simulink model "MRAClecture"  (R2022a)
settings: Solver=VariableStepAuto  StartTime=0.0  StopTime=100  RelTol=1e-3
undefined symbols (not defined in the file): a, a_m, b, b_m, c
settings Model: Creator=edgar  LastModifiedBy=edgar

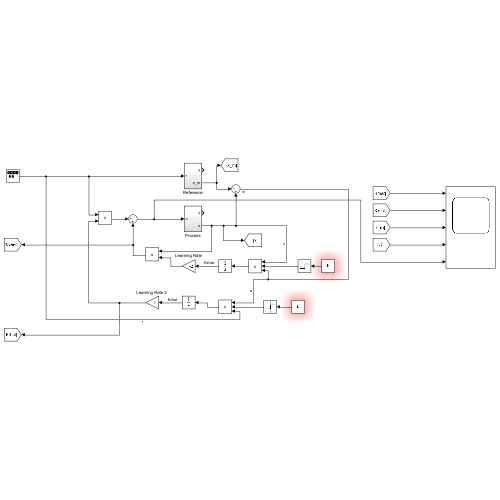
[thumbnail: Simulink's stored preview of the top-level diagram]
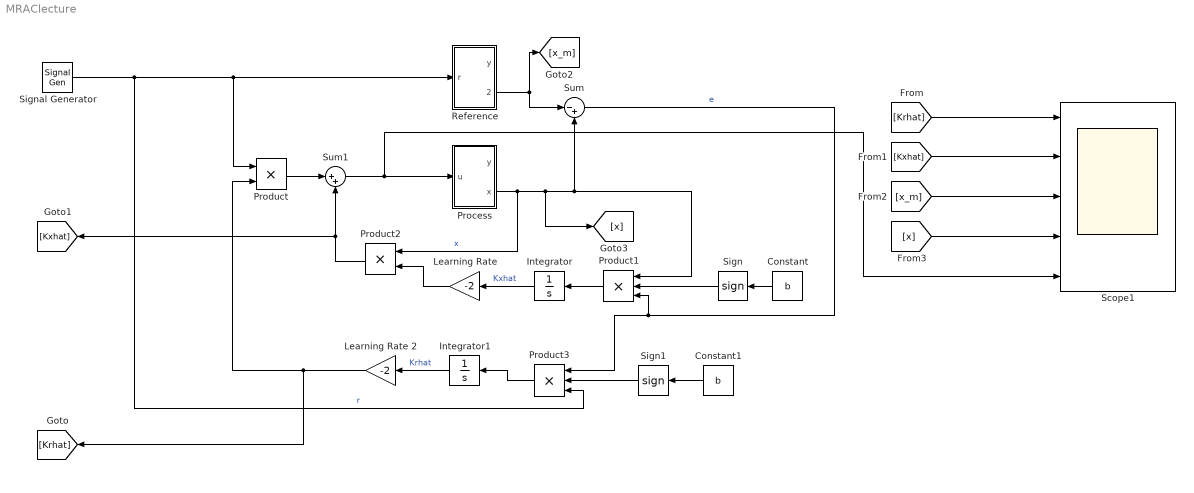
== system MRAClecture ==
  Constant : Constant  Value=b
  Constant1 : Constant  Value=b
  Integrator : Integrator
  Integrator1 : Integrator
  Learning Rate : Gain  Gain=-2
  "Learning Rate 2 " : Gain  Gain=-2
  Process : Subsystem
  Product : Product
  Product1 : Product  Inputs=3
  Product2 : Product
  Product3 : Product  Inputs=3
  Reference : Subsystem
  Scope1 : Scope  NumInputPorts=5
  Sign : Signum
  Sign1 : Signum
  Signal Generator : SignalGenerator  WaveForm=square  Frequency=0.2  Units=rad/sec
  Sum : Sum  Inputs=|-+
  Sum1 : Sum  Inputs=|++
  wires:
  Reference/2(x_m) -> [x_m], Sum/1
  Signal Generator/1 -> Product3/3, Reference/1(r), Product/1  "r"
  Sum1/1 -> Scope1/5, Process/1(u)
  Process/2(x) -> Product2/1, [x], Product1/1, Sum/2  "x"
  Product/1 -> Sum1/1
  Constant/1 -> Sign/1
  Product1/1 -> Integrator/1
  Integrator/1 -> Learning Rate/1  "Kxhat"
  Learning Rate/1 -> Product2/2
  Constant1/1 -> Sign1/1
  Integrator1/1 -> "Learning Rate 2 "/1  "Krhat"
  Product3/1 -> Integrator1/1
  "Learning Rate 2 "/1 -> [Krhat], Product/2
  Product2/1 -> [Kxhat], Sum1/2
  Sign/1 -> Product1/2
  Sum/1 -> Product3/1, Product1/3  "e"
  Sign1/1 -> Product3/2
  [Krhat] -> Scope1/1
  [Kxhat] -> Scope1/2
  [x_m] -> Scope1/3
  [x] -> Scope1/4

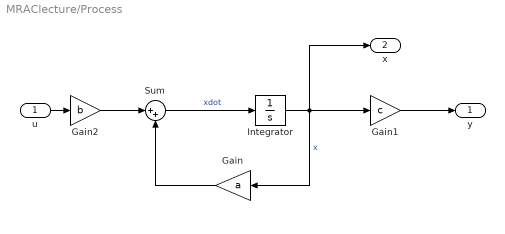
== system MRAClecture/Process ==
  u : Inport
  Gain : Gain  Gain=a
  Gain1 : Gain  Gain=c
  Gain2 : Gain  Gain=b
  Integrator : Integrator
  Sum : Sum  Inputs=|++
  y : Outport
  x : Outport  Port=2
  wires:
  Sum/1 -> Integrator/1  "xdot"
  Integrator/1 -> x/1, Gain1/1, Gain/1  "x"
  Gain1/1 -> y/1
  Gain2/1 -> Sum/1
  Gain/1 -> Sum/2
  u/1 -> Gain2/1

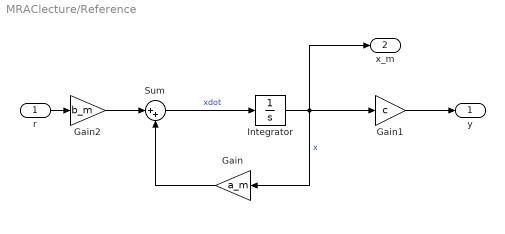
== system MRAClecture/Reference ==
  r : Inport
  Gain : Gain  Gain=a_m
  Gain1 : Gain  Gain=c
  Gain2 : Gain  Gain=b_m
  Integrator : Integrator
  Sum : Sum  Inputs=|++
  y : Outport
  x_m : Outport  Port=2
  wires:
  Sum/1 -> Integrator/1  "xdot"
  Integrator/1 -> x_m/1, Gain1/1, Gain/1  "x"
  Gain1/1 -> y/1
  Gain2/1 -> Sum/1
  Gain/1 -> Sum/2
  r/1 -> Gain2/1
